simulink model "lab_readyDIGIT2"  (R2020b)
settings: Solver=ode4  StartTime=0.0  StopTime=5  FixedStep=0.001  RelTol=1e-3
values from neighbouring files (symbols this model uses):
  degs2rpm = 0.166666666667    [DIGIT1-BE10.mat]    (also in DIGIT1-FE10.mat; DIGIT1-FE20.mat; DIGIT1-FE4.mat; DIGIT1-TR10.mat)
  denF = [1 0.515887399724 0.219018124689]    [DIGIT1-BE10.mat]    (also in DIGIT1-FE10.mat; DIGIT1-FE20.mat = [1 1.15847990004 0.419704605826]; DIGIT1-FE4.mat = [1 -0.53010968182 0.221694090774]; DIGIT1-TR10.mat)
  drv =     [DIGIT1-BE10.mat]    (also in DIGIT1-FE10.mat; DIGIT1-FE20.mat; DIGIT1-FE4.mat; DIGIT1-TR10.mat)
  filt =     [DIGIT1-BE10.mat]    (also in DIGIT1-FE10.mat; DIGIT1-FE20.mat; DIGIT1-FE4.mat; DIGIT1-TR10.mat)
  numF = [86.7452762207 0 -86.7452762207]    [DIGIT1-BE10.mat]    (also in DIGIT1-FE10.mat; DIGIT1-FE20.mat = [64.4546126467 0 -64.4546126467]; DIGIT1-FE4.mat = [86.4480511192 0 -86.4480511192]; DIGIT1-TR10.mat)
  rpm2rads = 0.10471975512    [DIGIT1-BE10.mat]    (also in DIGIT1-FE10.mat; DIGIT1-FE20.mat; DIGIT1-FE4.mat; DIGIT1-TR10.mat)
  sens =     [DIGIT1-BE10.mat]    (also in DIGIT1-FE10.mat; DIGIT1-FE20.mat; DIGIT1-FE4.mat; DIGIT1-TR10.mat)
  Ts = 0.01    [DIGIT1-BE10.mat]    (also in DIGIT1-FE10.mat; DIGIT1-FE20.mat = 0.02; DIGIT1-FE4.mat = 0.004; DIGIT1-TR10.mat)
undefined symbols (not defined in the file or in its folder): DiscIntNeverNeededParam, National_Instruments, PCI
libraries: sldrtlib x3
settings Model: ExtModeTrigDuration=50001  Creator=verrimarco  LastModifiedBy=verrimarco
settings DataIOCC: SaveFormat=StructureWithTime  InspectSignalLogs=on  ReturnWorkspaceOutputs=off  LoggingFileName=out.mat2
settings RTWCC: Description=Simulink Desktop Real-Time  SystemTargetFile=sldrt.tlc  TemplateMakefile=sldrt.tmf  RTWCompilerOptimization=on
settings CodeAppCC: MaxIdLength=95
settings SimulinkDesktopRealTimeCC: TargetPreCompLibLocation=C:\Program Files\MATLAB\R2020b\toolbox\sldrt\lib\win64

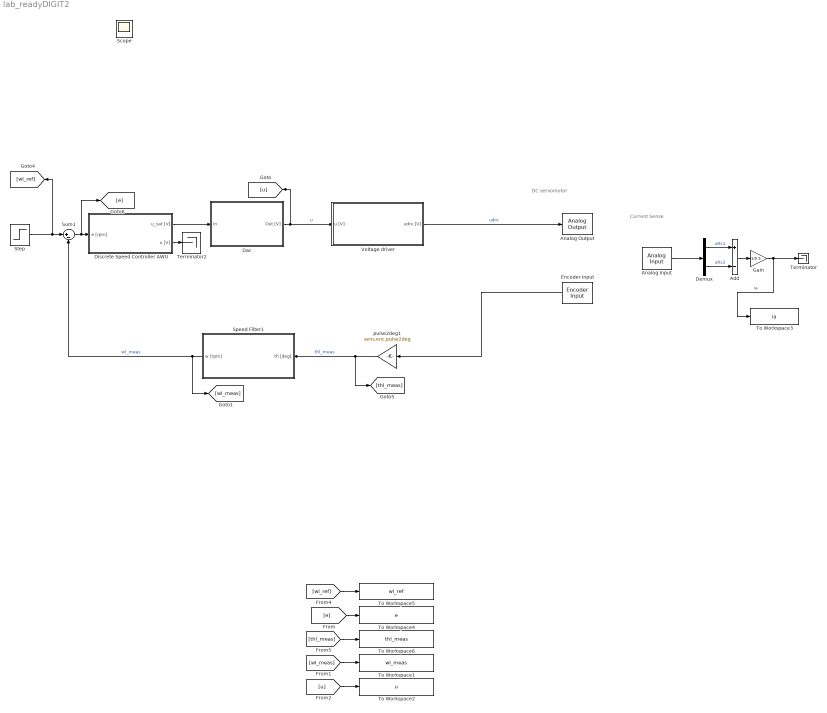
== system lab_readyDIGIT2 ==
  note: DC servomotor
  note: Current Sense
  Add : Sum  Inputs=+-
  Analog Input : sldrtlib/Analog Input  SampleTime=-1  MaxMissedTicks=10  ShowMissedTicks=off  YieldWhenWaiting=off  DrvName=National_Instruments/PCI-6221  DrvAddress=4294967295  DrvOptions=[0 0 0 2 0]  Channels=[1,2]  RangeMode=1  VoltRange=1  DataType=1
      settings: AttributesFormatString=National Instruments\nPCI-6221 [auto]
  Analog Output : sldrtlib/Analog Output  SampleTime=-1  MaxMissedTicks=10  ShowMissedTicks=off  YieldWhenWaiting=off  DrvName=National_Instruments/PCI-6221  DrvAddress=4294967295  DrvOptions=[0 0 0 2 0]  Channels=1  RangeMode=1  VoltRange=1  InitialValue=0  FinalValue=0
      settings: AttributesFormatString=National Instruments\nPCI-6221 [auto]
  Dac : Subsystem
  Demux : Demux  Outputs=2
  Discrete Speed Controller AWU : Subsystem
  Encoder Input : sldrtlib/Encoder Input  SampleTime=-1  MaxMissedTicks=10  ShowMissedTicks=off  YieldWhenWaiting=on  DrvName=National_Instruments/PCI-6221  DrvAddress=4294967295  DrvOptions=[0 0 0 2 0]  Channels=1  QuadMode=3  IndexPulse=1  InputFilter=Inf  DataType=1
      settings: AttributesFormatString=National Instruments\nPCI-6221 [auto]
  Gain : Gain  Gain=1/0.5
  Speed Filter1 : Subsystem
  Step : Step  After=250  SampleTime=0
  Sum1 : Sum  Inputs=|+-
  Terminator : Terminator
  Terminator2 : Terminator
  To Workspace1 : ToWorkspace  VariableName=wl_meas  SaveFormat=Structure With Time  SampleTime=-1
      settings: Save2DSignal=2-D array (concatenate along first dimension)
  To Workspace2 : ToWorkspace  VariableName=u  SaveFormat=Structure With Time  SampleTime=-1
      settings: Save2DSignal=2-D array (concatenate along first dimension)
  To Workspace3 : ToWorkspace  VariableName=ia  SaveFormat=Structure With Time  SampleTime=-1
  To Workspace4 : ToWorkspace  VariableName=e  SaveFormat=Structure With Time  SampleTime=-1
      settings: Save2DSignal=2-D array (concatenate along first dimension)
  To Workspace5 : ToWorkspace  VariableName=wl_ref  SaveFormat=Structure With Time  SampleTime=-1
      settings: Save2DSignal=2-D array (concatenate along first dimension)
  To Workspace6 : ToWorkspace  VariableName=thl_meas  SaveFormat=Structure With Time  SampleTime=-1
      settings: Save2DSignal=2-D array (concatenate along first dimension)
  Voltage driver : Subsystem
  pulse2deg1 : Gain  Gain=sens.enc.pulse2deg
  Scope : Scope
  wires:
  Analog Input/1 -> Demux/1
  Demux/1 -> Add/1  "uRs1"
  Demux/2 -> Add/2  "uRs2"
  Add/1 -> Gain/1
  Gain/1 -> To Workspace3/1, Terminator/1  "ia"
  Encoder Input/1 -> pulse2deg1/1
  [wl_ref] -> To Workspace5/1
  [wl_meas] -> To Workspace1/1
  [u] -> To Workspace2/1
  [thl_meas] -> To Workspace6/1
  [e] -> To Workspace4/1
  pulse2deg1/1 -> [thl_meas], Speed Filter1/1(th [deg])  "thl_meas"
  Discrete Speed Controller AWU/2(u [V]) -> Terminator2/1
  Dac/1(Out [V]) -> [u], Voltage driver/1(u [V])  "u"
  Discrete Speed Controller AWU/1(u_sat [V]) -> Dac/1(In)
  Sum1/1 -> [e], Discrete Speed Controller AWU/1(e [rpm])
  Voltage driver/1(udrv [V]) -> Analog Output/1  "udrv"
  Speed Filter1/1(w [rpm]) -> [wl_meas], Sum1/2  "wl_meas"
  Step/1 -> [wl_ref], Sum1/1

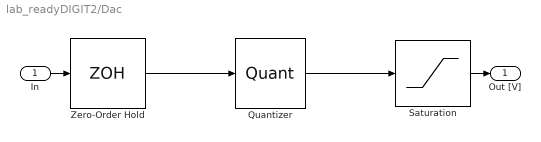
== system lab_readyDIGIT2/Dac ==
  In : Inport
  Quantizer : Quantizer  QuantizationInterval=daq.dac.q
  Saturation : Saturate  UpperLimit=10  LowerLimit=-10
  Zero-Order Hold : ZeroOrderHold  SampleTime=0.001
  Out [V] : Outport
  wires:
  In/1 -> Zero-Order Hold/1
  Zero-Order Hold/1 -> Quantizer/1
  Saturation/1 -> Out [V]/1
  Quantizer/1 -> Saturation/1

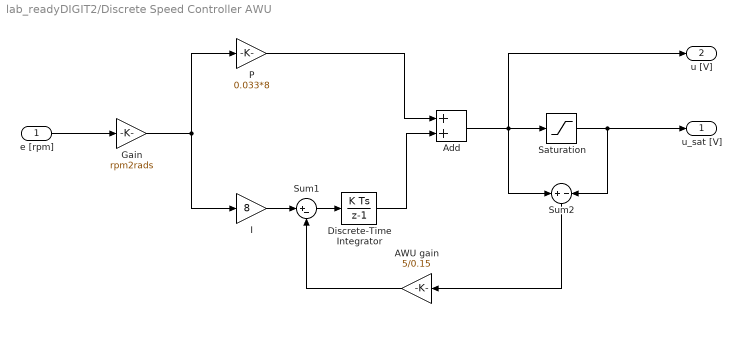
== system lab_readyDIGIT2/Discrete Speed Controller AWU ==
  e [rpm] : Inport
  AWU gain : Gain  Gain=5/0.15
  Add : Sum
  Discrete-Time Integrator : DiscreteIntegrator  SampleTime=Ts  ICPrevOutput=DiscIntNeverNeededParam  ICPrevScaledInput=DiscIntNeverNeededParam
  Gain : Gain  Gain=rpm2rads
  I : Gain  Gain=8
  P : Gain  Gain=0.033*8
  Saturation : Saturate  UpperLimit=10  LowerLimit=-10
  Sum1 : Sum  Inputs=|+-
  Sum2 : Sum  Inputs=+-
  u_sat [V] : Outport
  u [V] : Outport  Port=2
  wires:
  e [rpm]/1 -> Gain/1
  P/1 -> Add/1
  Add/1 -> u [V]/1, Sum2/1, Saturation/1
  Saturation/1 -> Sum2/2, u_sat [V]/1
  Gain/1 -> I/1, P/1
  Sum1/1 -> Discrete-Time Integrator/1
  I/1 -> Sum1/1
  AWU gain/1 -> Sum1/2
  Sum2/1 -> AWU gain/1
  Discrete-Time Integrator/1 -> Add/2

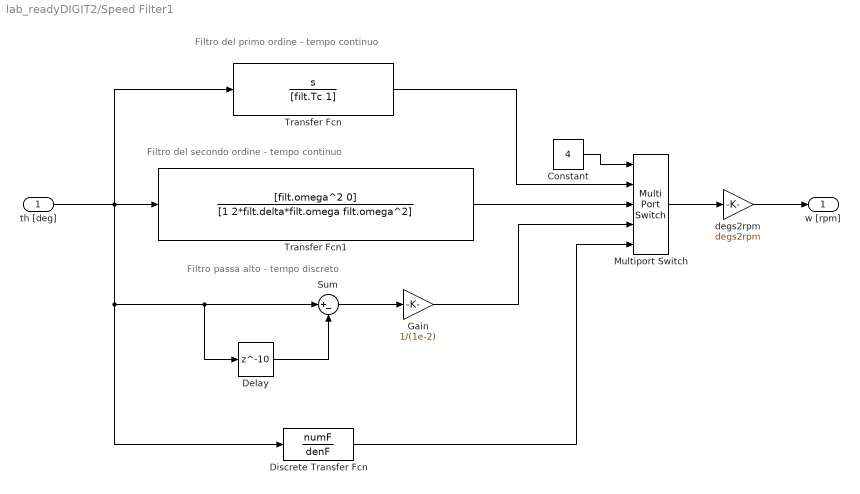
== system lab_readyDIGIT2/Speed Filter1 ==
  note: Filtro passa alto - tempo discreto
  note: Filtro del secondo ordine - tempo continuo
  note: Filtro del primo ordine - tempo continuo
  th [deg] : Inport
  Constant : Constant  Value=4
  Delay : Delay  DelayLength=10  InitialCondition=0
  Discrete Transfer Fcn : DiscreteTransferFcn  Numerator=numF  Denominator=denF  SampleTime=Ts
  Gain : Gain  Gain=1/(1e-2)
  Multiport Switch : MultiPortSwitch  Inputs=4
  Sum : Sum  Inputs=|+-
  Transfer Fcn : TransferFcn  Numerator=[1 0]  Denominator=[filt.Tc 1]
  Transfer Fcn1 : TransferFcn  Numerator=[filt.omega^2 0]  Denominator=[1 2*filt.delta*filt.omega filt.omega^2]
  degs2rpm : Gain  Gain=degs2rpm
  w [rpm] : Outport
  wires:
  degs2rpm/1 -> w [rpm]/1
  Transfer Fcn1/1 -> Multiport Switch/3
  Multiport Switch/1 -> degs2rpm/1
  Gain/1 -> Multiport Switch/4
  Delay/1 -> Sum/2
  Sum/1 -> Gain/1
  Constant/1 -> Multiport Switch/1
  Transfer Fcn/1 -> Multiport Switch/2
  th [deg]/1 -> Discrete Transfer Fcn/1, Delay/1, Sum/1, Transfer Fcn/1, Transfer Fcn1/1
  Discrete Transfer Fcn/1 -> Multiport Switch/5

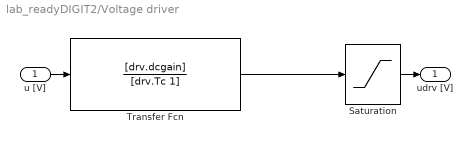
== system lab_readyDIGIT2/Voltage driver ==
  u [V] : Inport
  Saturation : Saturate  UpperLimit=12  LowerLimit=-12
  Transfer Fcn : TransferFcn  Numerator=[drv.dcgain]  Denominator=[drv.Tc 1]
  udrv [V] : Outport
  wires:
  u [V]/1 -> Transfer Fcn/1
  Saturation/1 -> udrv [V]/1
  Transfer Fcn/1 -> Saturation/1
